simulink model "partage_manoeuvreSV"  (Simulink 7.5)
settings: Solver=ode45  StartTime=0.0  StopTime=10.0  RelTol=1e-3
settings Model: Creator=paris  LastModifiedBy=paris

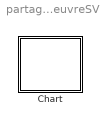
== system partage_manoeuvreSV ==
  Chart : Stateflow chart  TreatAsAtomicUnit=on

== stateflow chart Chart ==
  state MANOEUVRE_SV
    state DANS_VOIE
    state SORTIE_VOIE
      state SVG
        state HORS_VOIE
          state Recentration
          state Excentration
          MANOEUVRE_SV.SORTIE_VOIE.SVG.HORS_VOIE.Excentration -> MANOEUVRE_SV.SORTIE_VOIE.SVG.HORS_VOIE.Recentration : [ml.progression_SV==-1]
        state IMMINENTE
        MANOEUVRE_SV.SORTIE_VOIE.SVG.IMMINENTE -> MANOEUVRE_SV.SORTIE_VOIE.SVG.HORS_VOIE.Excentration : [ml.progression_SV==1]
        (default) -> MANOEUVRE_SV.SORTIE_VOIE.SVG.IMMINENTE : [ml.tlcCalcule<=1]
      state SVD
        state HORS_VOIE
          state Recentration
          state Excentration
          MANOEUVRE_SV.SORTIE_VOIE.SVD.HORS_VOIE.Excentration -> MANOEUVRE_SV.SORTIE_VOIE.SVD.HORS_VOIE.Recentration : [ml.progression_SV==-1]
        state IMMINENTE
        (default) -> MANOEUVRE_SV.SORTIE_VOIE.SVD.IMMINENTE : [ml.tlcCalcule<=1]
        MANOEUVRE_SV.SORTIE_VOIE.SVD.IMMINENTE -> MANOEUVRE_SV.SORTIE_VOIE.SVD.HORS_VOIE.Excentration : [ml.progression_SV==1]
    (default) -> DANS_VOIE
    MANOEUVRE_SV.SORTIE_VOIE.SVD.HORS_VOIE.Recentration -> DANS_VOIE : [ml.etat_SV==0]
    DANS_VOIE -> SVD [order 2] : [ml.lateralisation_SV==1]
    MANOEUVRE_SV.SORTIE_VOIE.SVG.HORS_VOIE.Recentration -> DANS_VOIE : [ml.etat_SV==0]
    DANS_VOIE -> SVG [order 1] : [ml.lateralisation_SV==-1]
